simulink model "tablerot"  (Simulink 7.5)
settings: Solver=FixedStepDiscrete  StartTime=0.0  StopTime=200.0  FixedStep=0.01  RelTol=1e-3
settings Model: Creator=avnish  LastModifiedBy=avnish
settings DataIOCC: MaxDataPoints=200000  SignalLoggingName=sigsOut
settings OptimizationCC: BlockReduction=off  BooleanDataType=off
settings DebuggingCC: SaveWithParameterizedLinksMsg=none  SignalResolutionControl=TryResolveAllWithWarning  SolverPrmCheckMsg=none  MultiTaskDSMMsg=warning  MultiTaskCondExecSysMsg=none  StrictBusMsg=None
settings HardwareCC: TargetUnknown=on
settings RTWCC: IncludeERTFirstTime=on

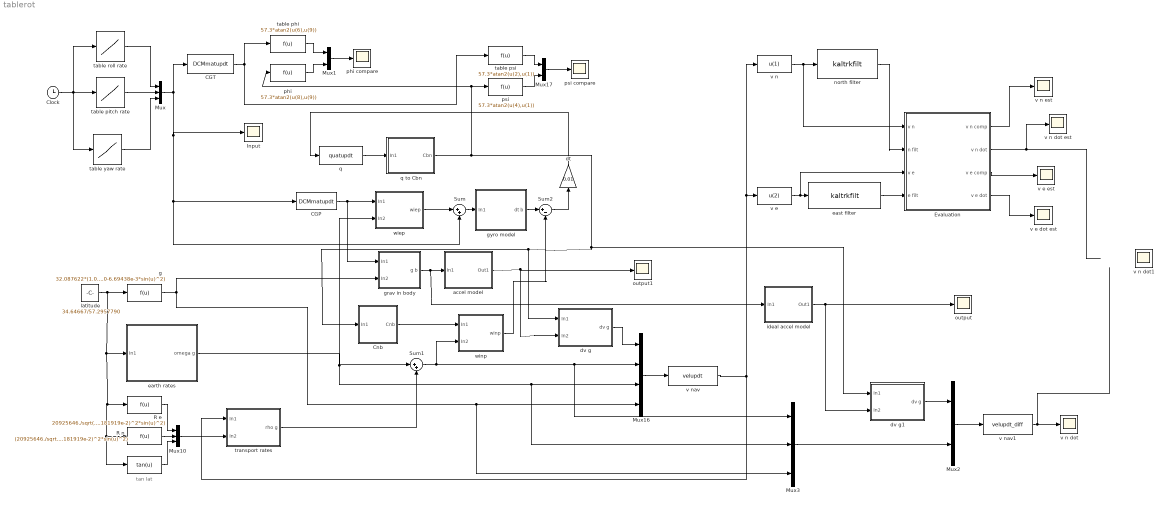
== system tablerot ==
  note: tan lat
  " " : Fcn  Expr=tan(u)
  CGP : S-Function  FunctionName=DCMmatupdt  Parameters=0.01,1,0,0,0,1,0,0,0,1  EnableBusSupport=off
  CGT : S-Function  FunctionName=DCMmatupdt  Parameters=0.01,1,0,0,0,1,0,0,0,1  EnableBusSupport=off
  Clock : Clock
      settings: Decimation=10
  Cnb : Subsystem
  Evaluation : Subsystem
  Input : Scope
      settings: TimeRange=200  YMin=0  YMax=0.16  SaveName=ScopeData6  MaxDataPoints=150000
  Mux : Mux  Inputs=3
  Mux1 : Mux  Inputs=2
  Mux10 : Mux  Inputs=3
  Mux16 : Mux
  Mux17 : Mux  Inputs=2
  Mux2 : Mux  Inputs=2
  Mux3 : Mux  Inputs=3
  R e : Fcn  Expr=20925646./sqrt(1.0-(8.181919e-2)^2*sin(u)^2)
  R n : Fcn  Expr=(20925646./sqrt(1.0-(8.181919e-2)^2*sin(u)^2))*(1.0-(8.181919e-2)^2)/(1.0-(8.181919e-2)^2*sin(u)^2)
  Sum : Sum  Inputs=|++  OutDataType=sfix(16)  OutScaling=2^0  SaturateOnIntegerOverflow=on  InputSameDT=on  OutDataTypeStr=Inherit: Same as first input
  Sum1 : Sum  Inputs=|++  OutDataType=sfix(16)  OutScaling=2^0  SaturateOnIntegerOverflow=on  InputSameDT=on  OutDataTypeStr=Inherit: Same as first input
  Sum2 : Sum  Inputs=|+-  OutDataType=sfix(16)  OutScaling=2^0  SaturateOnIntegerOverflow=on  InputSameDT=on  OutDataTypeStr=Inherit: Same as first input
  accel model : Subsystem
  dt : Gain  Gain=0.01  ParameterDataType=sfix(16)  ParameterScaling=2^0  OutDataType=sfix(16)  OutScaling=2^0  SaturateOnIntegerOverflow=on  OutDataTypeStr=Inherit: Same as input  ParamDataTypeStr=Inherit: Same as input
  dv g : Subsystem
  dv g1 : Subsystem
  earth rates : Subsystem
  east filter : S-Function  FunctionName=kaltrkfilt  Parameters=0.01,0.01,0.01,1.0,0.1,0.01  EnableBusSupport=off
  g : Fcn  Expr=32.087622*(1.0+1.93185e-3*sin(u)^2)/sqrt(1.0-6.69438e-3*sin(u)^2)
  grav in body : Subsystem
  gyro model : Subsystem
  ideal accel model : Subsystem
  latitude : Constant  Value=34.64667/57.2957790  OutDataType=sfix(16)  OutScaling=2^0
  north filter : S-Function  FunctionName=kaltrkfilt  Parameters=0.01,0.01,0.01,1.0,0.1,0.01  EnableBusSupport=off
  output : Scope
      settings: TimeRange=200  YMin=-1.4  YMax=0.3999999999999999  SaveName=ScopeData7  MaxDataPoints=150000
  output1 : Scope
      settings: TimeRange=200  YMin=-1.4  YMax=0.3999999999999999  SaveName=ScopeData8  MaxDataPoints=150000
  phi : Fcn  Expr=57.3*atan2(u(8),u(9))
  phi compare : Scope
      settings: TimeRange=200  YMin=-200  YMax=200  MaxDataPoints=150000
  psi : Fcn  Expr=57.3*atan2(u(4),u(1))
  psi compare : Scope
      settings: TimeRange=200  YMin=-50  YMax=200  MaxDataPoints=150000
  q : S-Function  FunctionName=quatupdt  Parameters=0.01,0,0,0,1  EnableBusSupport=off
  q to Cbn : Subsystem
  table phi : Fcn  Expr=57.3*atan2(u(6),u(9))
  table pitch rate : Lookup  InputValues=[0,150]  Table=[0,0]  OutDataType=sfix(16)  OutScaling=2^0  SaturateOnIntegerOverflow=on
  table psi : Fcn  Expr=57.3*atan2(u(2),u(1))
  "table roll rate " : Lookup  InputValues=[0,4.99,5,24.99,25,29.99,30,49.99,50,150]  Table=[0,0,pi/20.0,pi/20.0,0,0,pi/20.0,pi/20.0,0,0]  OutDataType=sfix(16)  OutScaling=2^0  SaturateOnIntegerOverflow=on
  table yaw rate : Lookup  InputValues=[0,109.99,110,129.99,130,150]  Table=[0,0,pi/20.0,pi/20.0,0,0]  OutDataType=sfix(16)  OutScaling=2^0  SaturateOnIntegerOverflow=on
  transport rates : Subsystem
  v e : Fcn  Expr=u(2)
  v e dot est : Scope
      settings: TimeRange=200  YMin=-1.4  YMax=0.3999999999999999  SaveName=ScopeData5  MaxDataPoints=150000
  v e est : Scope
      settings: TimeRange=200  YMin=-150  YMax=50  SaveName=ScopeData4  MaxDataPoints=150000
  v n : Fcn  Expr=u(1)
  v n dot : Scope
      settings: TimeRange=200  YMin=-0.8  YMax=0.6000000000000001  SaveName=ScopeData9  MaxDataPoints=150000
  v n dot est : Scope
      settings: TimeRange=200  YMin=-0.8  YMax=0.6000000000000001  SaveName=ScopeData3  MaxDataPoints=150000
  v n dot1 : Scope
      settings: TimeRange=200  YMin=-0.8  YMax=0.6000000000000001  SaveName=ScopeData10  MaxDataPoints=150000
  v n est : Scope
      settings: TimeRange=200  YMin=950  YMax=1650  SaveName=ScopeData2  MaxDataPoints=150000
  v nav : S-Function  FunctionName=velupdt  Parameters=0.01,0,0,0  EnableBusSupport=off
  v nav1 : S-Function  FunctionName=velupdt_diff  Parameters=0.01,0,0,0  EnableBusSupport=off
  wiep : Subsystem
  winp : Subsystem
  wires:
  Clock/1 -> table pitch rate/1, "table roll rate "/1, table yaw rate/1
  table pitch rate/1 -> Mux/2
  Mux/1 -> CGT/1, CGP/1, Sum/2, Input/1
  latitude/1 -> g/1, R e/1, R n/1, " "/1, earth rates/1(In1)
  Mux1/1 -> phi compare/1
  CGP/1 -> grav in body/1(In1), wiep/1(In1)
  earth rates/1(omega g) -> Sum1/1, wiep/2(In2), Mux16/3, Mux3/2
  g/1 -> grav in body/2(In2), Mux16/4, Mux3/3
  R e/1 -> Mux10/1
  R n/1 -> Mux10/2
  " "/1 -> Mux10/3
  Mux10/1 -> transport rates/2(In2)
  transport rates/1(rho g) -> Sum1/2
  q to Cbn/1(Cbn) -> psi/1, phi/1, Cnb/1(In1), dv g/1(In1), dv g1/1(In1)
  Mux16/1 -> v nav/1
  v nav/1 -> transport rates/1(In1), v n/1, v e/1
  CGT/1 -> table phi/1, table psi/1
  phi/1 -> Mux1/2
  Mux17/1 -> psi compare/1
  table psi/1 -> Mux17/1
  psi/1 -> Mux17/2
  wiep/1(wiep) -> Sum/1
  winp/1(winp) -> Sum2/2
  accel model/1(Out1) -> output1/1, dv g/2(In2)
  gyro model/1(dt b) -> Sum2/1
  "table roll rate "/1 -> Mux/1
  table yaw rate/1 -> Mux/3
  v n/1 -> north filter/1, Evaluation/1(v n)
  Evaluation/1(v n comp) -> v n est/1
  Evaluation/2(v n dot) -> v n dot est/1
  v e/1 -> east filter/1, Evaluation/3(v e)
  Evaluation/3(v e comp) -> v e est/1
  north filter/1 -> Evaluation/2(n filt)
  east filter/1 -> Evaluation/4(e filt)
  Sum2/1 -> dt/1
  dt/1 -> q/1
  Cnb/1(Cnb) -> winp/1(In1)
  Sum/1 -> gyro model/1(In1)
  grav in body/1(g b) -> accel model/1(In1), ideal accel model/1(In1)
  q/1 -> q to Cbn/1(In1)
  Evaluation/4(v e dot) -> v e dot est/1
  dv g/1(dv g) -> Mux16/1
  Sum1/1 -> winp/2(In2), Mux16/2, Mux3/1
  table phi/1 -> Mux1/1
  ideal accel model/1(Out1) -> output/1, dv g1/2(In2)
  dv g1/1(dv g) -> Mux2/1
  Mux3/1 -> Mux2/2
  Mux2/1 -> v nav1/1
  v nav1/1 -> v n dot/1
  ? -> v n dot1/1

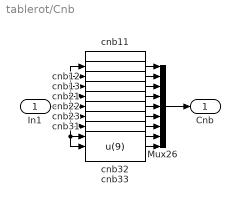
== system tablerot/Cnb ==
  In1 : Inport  OutDataType=sfix(16)  OutScaling=2^0
  Mux26 : Mux  Inputs=9
  cnb11 : Fcn  Expr=u(1)
  cnb12 : Fcn  Expr=u(4)
  cnb13 : Fcn  Expr=u(7)
  cnb21 : Fcn  Expr=u(2)
  cnb22 : Fcn  Expr=u(5)
  cnb23 : Fcn  Expr=u(8)
  cnb31 : Fcn  Expr=u(3)
  cnb32 : Fcn  Expr=u(6)
  cnb33 : Fcn  Expr=u(9)
  Cnb : Outport
  wires:
  cnb11/1 -> Mux26/1
  cnb12/1 -> Mux26/2
  cnb13/1 -> Mux26/3
  cnb21/1 -> Mux26/4
  cnb22/1 -> Mux26/5
  cnb23/1 -> Mux26/6
  cnb31/1 -> Mux26/7
  cnb32/1 -> Mux26/8
  cnb33/1 -> Mux26/9
  In1/1 -> cnb21/1, cnb13/1, cnb12/1, cnb11/1, cnb22/1, cnb23/1, cnb32/1, cnb33/1, cnb31/1
  Mux26/1 -> Cnb/1

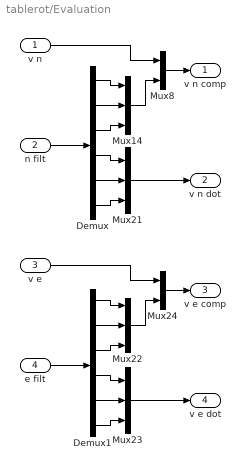
== system tablerot/Evaluation ==
  v n : Inport  OutDataType=sfix(16)  OutScaling=2^0
  n filt : Inport  Port=2  OutDataType=sfix(16)  OutScaling=2^0
  v e : Inport  Port=3  OutDataType=sfix(16)  OutScaling=2^0
  e filt : Inport  Port=4  OutDataType=sfix(16)  OutScaling=2^0
  Demux : Demux  Outputs=6
  Demux1 : Demux  Outputs=6
  Mux{14,21..23} (4 alike) : Mux  Inputs=3
  Mux24 : Mux  Inputs=2
  Mux8 : Mux  Inputs=2
  v n comp : Outport
  v n dot : Outport  Port=2
  v e comp : Outport  Port=3
  v e dot : Outport  Port=4
  wires:
  Mux14/1 -> Mux8/2
  Mux22/1 -> Mux24/2
  Demux/1 -> Mux14/1
  Demux/2 -> Mux14/2
  Demux/3 -> Mux14/3
  Demux/4 -> Mux21/1
  Demux/5 -> Mux21/2
  Demux/6 -> Mux21/3
  Demux1/3 -> Mux22/3
  Demux1/4 -> Mux23/1
  Demux1/5 -> Mux23/2
  Demux1/6 -> Mux23/3
  Demux1/2 -> Mux22/2
  Demux1/1 -> Mux22/1
  v n/1 -> Mux8/1
  Mux8/1 -> v n comp/1
  n filt/1 -> Demux/1
  Mux21/1 -> v n dot/1
  v e/1 -> Mux24/1
  Mux24/1 -> v e comp/1
  e filt/1 -> Demux1/1
  Mux23/1 -> v e dot/1

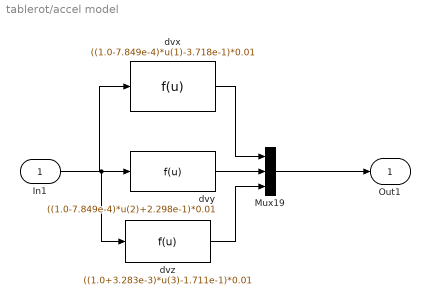
== system tablerot/accel model ==
  In1 : Inport  OutDataType=sfix(16)  OutScaling=2^0
  Mux19 : Mux  Inputs=3
  dvx : Fcn  Expr=((1.0-7.849e-4)*u(1)-3.718e-1)*0.01
  dvy : Fcn  Expr=((1.0-7.849e-4)*u(2)+2.298e-1)*0.01
  dvz : Fcn  Expr=((1.0+3.283e-3)*u(3)-1.711e-1)*0.01
  Out1 : Outport
  wires:
  In1/1 -> dvy/1, dvx/1, dvz/1
  Mux19/1 -> Out1/1
  dvx/1 -> Mux19/1
  dvy/1 -> Mux19/2
  dvz/1 -> Mux19/3

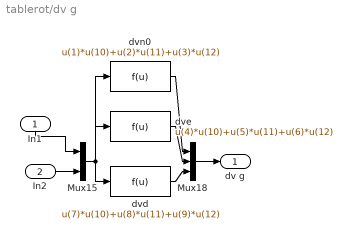
== system tablerot/dv g ==
  In1 : Inport  OutDataType=sfix(16)  OutScaling=2^0
  In2 : Inport  Port=2  OutDataType=sfix(16)  OutScaling=2^0
  Mux15 : Mux  Inputs=2
  Mux18 : Mux  Inputs=3
  dvd : Fcn  Expr=u(7)*u(10)+u(8)*u(11)+u(9)*u(12)
  dve : Fcn  Expr=u(4)*u(10)+u(5)*u(11)+u(6)*u(12)
  dvn0 : Fcn  Expr=u(1)*u(10)+u(2)*u(11)+u(3)*u(12)
  dv g : Outport
  wires:
  Mux15/1 -> dve/1, dvn0/1, dvd/1
  dve/1 -> Mux18/2
  dvn0/1 -> Mux18/1
  dvd/1 -> Mux18/3
  In1/1 -> Mux15/1
  Mux18/1 -> dv g/1
  In2/1 -> Mux15/2

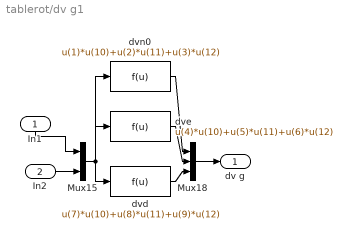
== system tablerot/dv g1 ==
  In1 : Inport  OutDataType=sfix(16)  OutScaling=2^0
  In2 : Inport  Port=2  OutDataType=sfix(16)  OutScaling=2^0
  Mux15 : Mux  Inputs=2
  Mux18 : Mux  Inputs=3
  dvd : Fcn  Expr=u(7)*u(10)+u(8)*u(11)+u(9)*u(12)
  dve : Fcn  Expr=u(4)*u(10)+u(5)*u(11)+u(6)*u(12)
  dvn0 : Fcn  Expr=u(1)*u(10)+u(2)*u(11)+u(3)*u(12)
  dv g : Outport
  wires:
  In2/1 -> Mux15/2
  Mux18/1 -> dv g/1
  In1/1 -> Mux15/1
  dvd/1 -> Mux18/3
  dvn0/1 -> Mux18/1
  dve/1 -> Mux18/2
  Mux15/1 -> dvd/1, dvn0/1, dve/1

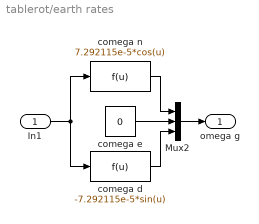
== system tablerot/earth rates ==
  In1 : Inport  OutDataType=sfix(16)  OutScaling=2^0
  Mux2 : Mux  Inputs=3
  comega d : Fcn  Expr=-7.292115e-5*sin(u)
  comega e : Constant  Value=0  OutDataType=sfix(16)  OutScaling=2^0
  comega n : Fcn  Expr=7.292115e-5*cos(u)
  omega g : Outport
  wires:
  comega n/1 -> Mux2/1
  comega e/1 -> Mux2/2
  comega d/1 -> Mux2/3
  In1/1 -> comega n/1, comega d/1
  Mux2/1 -> omega g/1

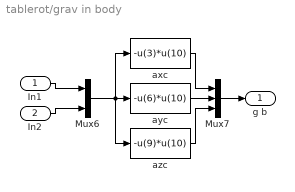
== system tablerot/grav in body ==
  In1 : Inport  OutDataType=sfix(16)  OutScaling=2^0
  In2 : Inport  Port=2  OutDataType=sfix(16)  OutScaling=2^0
  Mux6 : Mux  Inputs=2
  Mux7 : Mux  Inputs=3
  axc : Fcn  Expr=-u(3)*u(10)
  ayc : Fcn  Expr=-u(6)*u(10)
  azc : Fcn  Expr=-u(9)*u(10)
  g b : Outport
  wires:
  Mux6/1 -> ayc/1, axc/1, azc/1
  ayc/1 -> Mux7/2
  axc/1 -> Mux7/1
  azc/1 -> Mux7/3
  In1/1 -> Mux6/1
  Mux7/1 -> g b/1
  In2/1 -> Mux6/2

== system tablerot/gyro model ==
  In1 : Inport  OutDataType=sfix(16)  OutScaling=2^0
  Mux20 : Mux  Inputs=3
  dgx : Fcn  Expr=((1.0-3.805718e-3)*u(1)+1.443327e-5)
  dgy : Fcn  Expr=((1.0-3.805718e-3)*u(2)+8.941422e-5)
  dgz : Fcn  Expr=((1.0-1.440145e-3)*u(3)+1.588867e-5)
  dt b : Outport
  wires:
  dgy/1 -> Mux20/2
  dgz/1 -> Mux20/3
  dgx/1 -> Mux20/1
  In1/1 -> dgx/1, dgz/1, dgy/1
  Mux20/1 -> dt b/1

== system tablerot/ideal accel model ==
  In1 : Inport  OutDataType=sfix(16)  OutScaling=2^0
  Mux19 : Mux  Inputs=3
  dvx : Fcn  Expr=(u(1))*0.01
  dvy : Fcn  Expr=(u(2))*0.01
  dvz : Fcn  Expr=(u(3))*0.01
  Out1 : Outport
  wires:
  dvz/1 -> Mux19/3
  dvy/1 -> Mux19/2
  dvx/1 -> Mux19/1
  Mux19/1 -> Out1/1
  In1/1 -> dvz/1, dvx/1, dvy/1

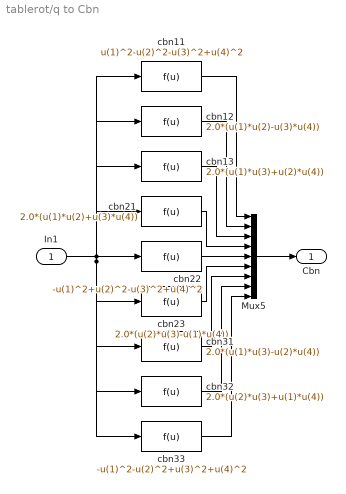
== system tablerot/q to Cbn ==
  In1 : Inport  OutDataType=sfix(16)  OutScaling=2^0
  Mux5 : Mux  Inputs=9
  cbn11 : Fcn  Expr=u(1)^2-u(2)^2-u(3)^2+u(4)^2
  cbn12 : Fcn  Expr=2.0*(u(1)*u(2)-u(3)*u(4))
  cbn13 : Fcn  Expr=2.0*(u(1)*u(3)+u(2)*u(4))
  cbn21 : Fcn  Expr=2.0*(u(1)*u(2)+u(3)*u(4))
  cbn22 : Fcn  Expr=-u(1)^2+u(2)^2-u(3)^2+u(4)^2
  cbn23 : Fcn  Expr=2.0*(u(2)*u(3)-u(1)*u(4))
  cbn31 : Fcn  Expr=2.0*(u(1)*u(3)-u(2)*u(4))
  cbn32 : Fcn  Expr=2.0*(u(2)*u(3)+u(1)*u(4))
  cbn33 : Fcn  Expr=-u(1)^2-u(2)^2+u(3)^2+u(4)^2
  Cbn : Outport
  wires:
  cbn11/1 -> Mux5/1
  cbn12/1 -> Mux5/2
  cbn13/1 -> Mux5/3
  cbn21/1 -> Mux5/4
  cbn22/1 -> Mux5/5
  cbn23/1 -> Mux5/6
  cbn31/1 -> Mux5/7
  cbn32/1 -> Mux5/8
  cbn33/1 -> Mux5/9
  In1/1 -> cbn11/1, cbn12/1, cbn13/1, cbn21/1, cbn22/1, cbn23/1, cbn31/1, cbn32/1, cbn33/1
  Mux5/1 -> Cbn/1

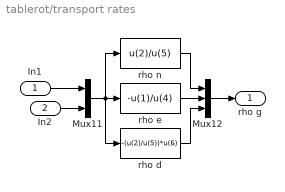
== system tablerot/transport rates ==
  In1 : Inport  OutDataType=sfix(16)  OutScaling=2^0
  In2 : Inport  Port=2  OutDataType=sfix(16)  OutScaling=2^0
  Mux11 : Mux  Inputs=2
  Mux12 : Mux  Inputs=3
  rho d : Fcn  Expr=-(u(2)/u(5))*u(6)
  rho e : Fcn  Expr=-u(1)/u(4)
  rho n : Fcn  Expr=u(2)/u(5)
  rho g : Outport
  wires:
  Mux11/1 -> rho n/1, rho e/1, rho d/1
  rho e/1 -> Mux12/2
  rho n/1 -> Mux12/1
  rho d/1 -> Mux12/3
  In1/1 -> Mux11/1
  Mux12/1 -> rho g/1
  In2/1 -> Mux11/2

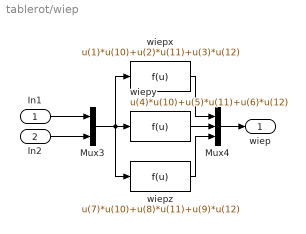
== system tablerot/wiep ==
  In1 : Inport  OutDataType=sfix(16)  OutScaling=2^0
  In2 : Inport  Port=2  OutDataType=sfix(16)  OutScaling=2^0
  Mux3 : Mux  Inputs=2
  Mux4 : Mux  Inputs=3
  wiepx : Fcn  Expr=u(1)*u(10)+u(2)*u(11)+u(3)*u(12)
  wiepy : Fcn  Expr=u(4)*u(10)+u(5)*u(11)+u(6)*u(12)
  wiepz : Fcn  Expr=u(7)*u(10)+u(8)*u(11)+u(9)*u(12)
  wiep : Outport
  wires:
  Mux3/1 -> wiepy/1, wiepz/1, wiepx/1
  wiepy/1 -> Mux4/2
  wiepx/1 -> Mux4/1
  wiepz/1 -> Mux4/3
  In1/1 -> Mux3/1
  Mux4/1 -> wiep/1
  In2/1 -> Mux3/2

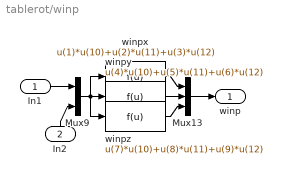
== system tablerot/winp ==
  In1 : Inport  OutDataType=sfix(16)  OutScaling=2^0
  In2 : Inport  Port=2  OutDataType=sfix(16)  OutScaling=2^0
  Mux13 : Mux  Inputs=3
  Mux9 : Mux  Inputs=2
  winpx : Fcn  Expr=u(1)*u(10)+u(2)*u(11)+u(3)*u(12)
  winpy : Fcn  Expr=u(4)*u(10)+u(5)*u(11)+u(6)*u(12)
  winpz : Fcn  Expr=u(7)*u(10)+u(8)*u(11)+u(9)*u(12)
  winp : Outport
  wires:
  Mux9/1 -> winpy/1, winpx/1, winpz/1
  winpy/1 -> Mux13/2
  winpx/1 -> Mux13/1
  winpz/1 -> Mux13/3
  In1/1 -> Mux9/1
  Mux13/1 -> winp/1
  In2/1 -> Mux9/2
